simulink library "receiver_sender"  (R2021a)
settings: Solver=ode45  StartTime=0.0  StopTime=10.0  RelTol=1e-3  EnableMultiTasking=on
libraries: dspnetwork x4, etargetslib x4
settings Model: Creator=Adriano  LastModifiedBy=hgu8
settings SolverCC: AlgebraicLoopSolver=TrustRegion
settings DataIOCC: LimitDataPoints=on  SaveFormat=Array  ReturnWorkspaceOutputs=off
settings OptimizationCC: LifeSpan=inf
settings DebuggingCC: UnderspecifiedInitializationDetection=Classic  MergeDetectMultiDrivingBlocksExec=none  SolverPrmCheckMsg=warning  StateNameClashWarn=warning  SFUnexpectedBacktrackingDiag=warning  SFNoUnconditionalDefaultTransitionDiag=warning  SFExecutionAtInitializationDiag=none  SFMachineParentedDataDiag=warning  ArithmeticOperatorsInVariantConditions=warning
settings HardwareCC: ProdBitPerPointer=32  ProdBitPerSizeT=32  ProdBitPerPtrDiffT=32  ProdLargestAtomicFloat=None  ProdIntDivRoundTo=Undefined  ProdEndianess=Unspecified  ProdWordSize=32  ProdHWDeviceType=32-bit Generic
settings ModelReferenceCC: PropagateSignalLabelsOutOfModel=off
settings SFSimCC: SimUseLocalCustomCode=off  CustomCodeUndefinedFunction=UseInterfaceOnly
settings RTWCC: RTWUseLocalCustomCode=off
settings CodeAppCC: StateflowObjectComments=on
settings GRTTargetCC: TargetLangStandard=C89/C90 (ANSI)
settings ConfigComp: CovMetricSettings=dw  CovSaveCumulativeToWorkspaceVar=on  CovSaveSingleToWorkspaceVar=on  CovExternalEMLEnable=off

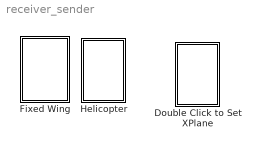
== system receiver_sender ==
  Double Click to Set XPlane : Subsystem
      settings: OpenFcn=selecting_parameters()
  Fixed Wing : Subsystem
  Helicopter : Subsystem

== system receiver_sender/Double Click to Set XPlane ==

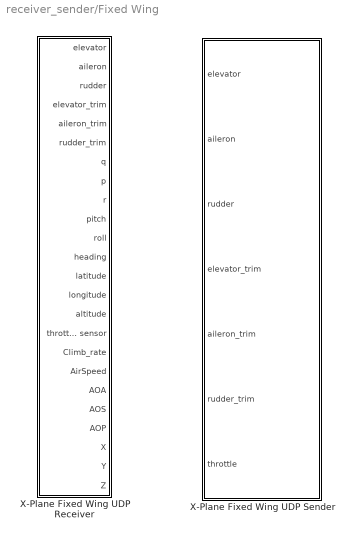
== system receiver_sender/Fixed Wing ==
  X-Plane Fixed Wing UDP Receiver : Subsystem  mask{ip_adress='127.0.0.1', port_number=49004}
      mask prompts: ip_adress "Local IP Adress (default: '127.0.0.1' )"; port_number "Output Port Number (defaut: '49004')"
      mask help: This block is configured to receiver data from a fixed wing aircraft on X-Plane Flight Simulator.
      mask Help: Contact adrianobittar@gmail.com
  X-Plane Fixed Wing UDP Sender : Subsystem  mask{ip_adress='127.0.0.1', port_number=49000}
      mask prompts: ip_adress "Local IP Adress (default: '127.0.0.1' )"; port_number "Output Port Number (defaut: '49000')"
      mask help: This block is configured to send data to a fixed wing aircraft on X-Plane Flight Simulator.
      mask Help: Contact adrianobittar@gmail.com

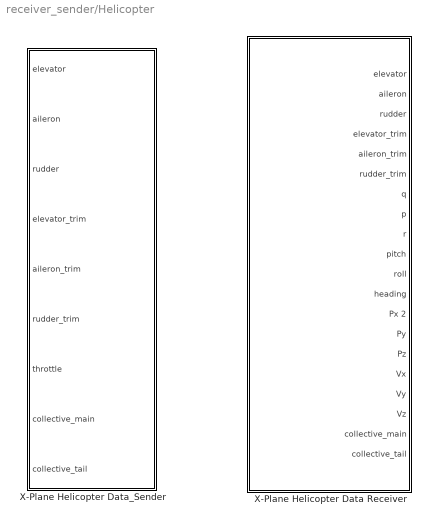
== system receiver_sender/Helicopter ==
  X-Plane Helicopter Data Receiver : Subsystem  AncestorBlock=DU2SRI_Heli_Sim/X-Plane Communication Blockset /X-Plane Data Receiver  mask{ip_adress='127.0.0.1', port_number=49004}
      mask prompts: ip_adress "Local IP Adress (default: '127.0.0.1')"; port_number "Input Port Number (default: '49004')"
      mask help: This block is configured to receive data to an helicopter aircraft on X-Plane Flight Simulator.
      mask Help: Contact adrianobittar@gmail.com
  X-Plane Helicopter Data_Sender : Subsystem  AncestorBlock=DU2SRI_Heli_Sim/X-Plane Communication Blockset /X-Plane Data_Sender  mask{ip_address='127.0.0.1', port_number=49000, max_col_main=12, min_col_main=0, max_col_tail=5, min_col_tail=-5}
      mask prompts: ip_address "Local IP Address (default: '127.0.0.1' )"; port_number "Output Port Number (defaut: '49000')"; max_col_main "Max Angle For Collective Main"; min_col_main "Min Angle For Collective Main"; max_col_tail "Max Angle For Collective Tail"; min_col_tail "Min Angle For Collective Tail"
      mask help: This block is configured to send data to an helicopter aircraft on X-Plane Flight Simulator.
      mask Help: contact adrianobittar@gmail.com

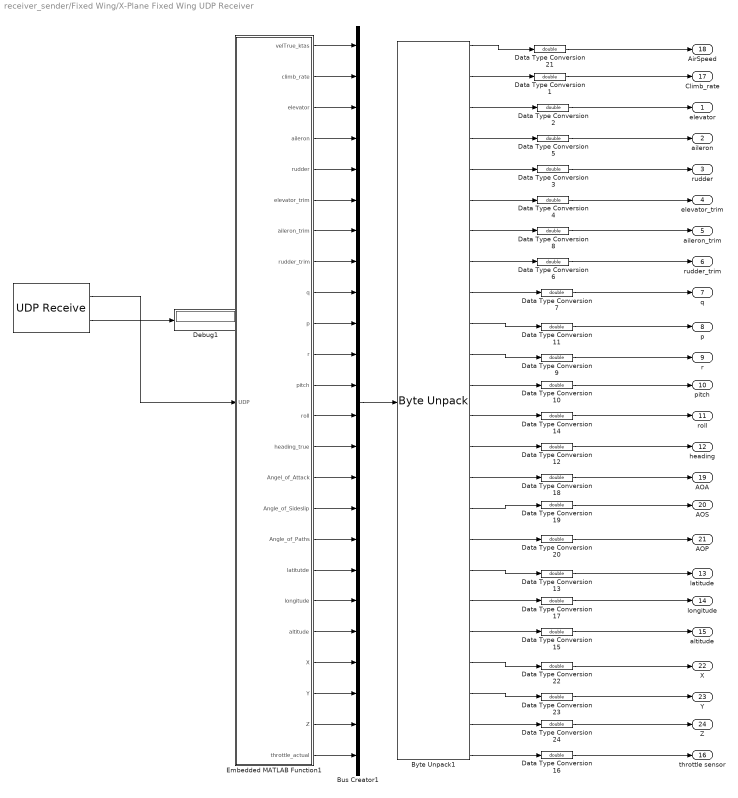
== system receiver_sender/Fixed Wing/X-Plane Fixed Wing UDP Receiver ==
  "    " : dspnetwork/UDP Receive  localURL='0.0.0.0'  localPort=port_number  remoteURL=ip_adress  remotePort=-1  recvBufferSize=8192  dims=500  signalDatatype=uint8  isComplex=off  isVarSize=off  showBlockingTime=on  blockingTime=20  sampletime=0.01  blockPlatform=WINDOWS
  Bus Creator1 : BusCreator  Inputs=24
  Byte Unpack1 : etargetslib/Byte Unpack  dimensions={1,1,1,1,1,1,1,1,1,1,1,1,1,1,1,1,1,1,1,1,1,1,1,1}  datatypes={'single','single','single','single','single','single','single','single','single','single','single','single','single','single','single','single','single','single','single','single','single','single','single','single'}  byteAlign=1
  Data Type Conversion{1..24} (24 alike) : DataTypeConversion  OutDataTypeStr=double  SaturateOnIntegerOverflow=on
  "Debug1 " : Display
  Embedded MATLAB Function1 : MATLAB Function  TreatAsAtomicUnit=on
  "elevator " : Outport
  aileron : Outport  Port=2
  rudder : Outport  Port=3
  elevator_trim : Outport  Port=4
  aileron_trim : Outport  Port=5
  rudder_trim : Outport  Port=6
  q : Outport  Port=7
  p : Outport  Port=8
  r : Outport  Port=9
  pitch : Outport  Port=10
  roll : Outport  Port=11
  heading : Outport  Port=12
  latitude : Outport  Port=13
  longitude : Outport  Port=14
  altitude : Outport  Port=15
  throttle sensor : Outport  Port=16
  Climb_rate : Outport  Port=17
  AirSpeed : Outport  Port=18
  AOA : Outport  Port=19
  AOS : Outport  Port=20
  AOP : Outport  Port=21
  X : Outport  Port=22
  Y : Outport  Port=23
  Z : Outport  Port=24
  wires:
  Data Type Conversion9/1 -> r/1
  Data Type Conversion10/1 -> pitch/1
  "    "/2 -> "Debug1 "/1
  Data Type Conversion21/1 -> AirSpeed/1
  Data Type Conversion1/1 -> Climb_rate/1
  Data Type Conversion2/1 -> "elevator "/1
  Data Type Conversion5/1 -> aileron/1
  Data Type Conversion8/1 -> aileron_trim/1
  Data Type Conversion3/1 -> rudder/1
  Data Type Conversion4/1 -> elevator_trim/1
  Data Type Conversion6/1 -> rudder_trim/1
  Data Type Conversion7/1 -> q/1
  Data Type Conversion12/1 -> heading/1
  Data Type Conversion13/1 -> latitude/1
  Data Type Conversion14/1 -> roll/1
  Data Type Conversion17/1 -> longitude/1
  Data Type Conversion15/1 -> altitude/1
  Data Type Conversion16/1 -> throttle sensor/1
  Data Type Conversion11/1 -> p/1
  Data Type Conversion18/1 -> AOA/1
  Data Type Conversion19/1 -> AOS/1
  Data Type Conversion20/1 -> AOP/1
  Data Type Conversion22/1 -> X/1
  Data Type Conversion23/1 -> Y/1
  Data Type Conversion24/1 -> Z/1
  "    "/1 -> Embedded MATLAB Function1/1(UDP)
  Embedded MATLAB Function1/1(velTrue_ktas) -> Bus Creator1/1
  Embedded MATLAB Function1/2(climb_rate) -> Bus Creator1/2
  Embedded MATLAB Function1/3(elevator) -> Bus Creator1/3
  Embedded MATLAB Function1/4(aileron) -> Bus Creator1/4
  Embedded MATLAB Function1/5(rudder) -> Bus Creator1/5
  Embedded MATLAB Function1/6(elevator_trim) -> Bus Creator1/6
  Embedded MATLAB Function1/7(aileron_trim) -> Bus Creator1/7
  Embedded MATLAB Function1/8(rudder_trim) -> Bus Creator1/8
  Embedded MATLAB Function1/9(q) -> Bus Creator1/9
  Embedded MATLAB Function1/10(p) -> Bus Creator1/10
  Embedded MATLAB Function1/11(r) -> Bus Creator1/11
  Embedded MATLAB Function1/12(pitch) -> Bus Creator1/12
  Embedded MATLAB Function1/13(roll) -> Bus Creator1/13
  Embedded MATLAB Function1/14(heading_true) -> Bus Creator1/14
  Embedded MATLAB Function1/15(Angel_of_Attack) -> Bus Creator1/15
  Embedded MATLAB Function1/16(Angle_of_Sideslip) -> Bus Creator1/16
  Embedded MATLAB Function1/17(Angle_of_Paths) -> Bus Creator1/17
  Embedded MATLAB Function1/18(latitutde) -> Bus Creator1/18
  Embedded MATLAB Function1/19(longitude) -> Bus Creator1/19
  Embedded MATLAB Function1/20(altitude) -> Bus Creator1/20
  Embedded MATLAB Function1/21(X) -> Bus Creator1/21
  Embedded MATLAB Function1/22(Y) -> Bus Creator1/22
  Embedded MATLAB Function1/23(Z) -> Bus Creator1/23
  Embedded MATLAB Function1/24(throttle_actual) -> Bus Creator1/24
  Bus Creator1/1 -> Byte Unpack1/1
  Byte Unpack1/1 -> Data Type Conversion21/1
  Byte Unpack1/2 -> Data Type Conversion1/1
  Byte Unpack1/3 -> Data Type Conversion2/1
  Byte Unpack1/4 -> Data Type Conversion5/1
  Byte Unpack1/5 -> Data Type Conversion3/1
  Byte Unpack1/6 -> Data Type Conversion4/1
  Byte Unpack1/7 -> Data Type Conversion8/1
  Byte Unpack1/8 -> Data Type Conversion6/1
  Byte Unpack1/9 -> Data Type Conversion7/1
  Byte Unpack1/10 -> Data Type Conversion11/1
  Byte Unpack1/11 -> Data Type Conversion9/1
  Byte Unpack1/12 -> Data Type Conversion10/1
  Byte Unpack1/13 -> Data Type Conversion14/1
  Byte Unpack1/14 -> Data Type Conversion12/1
  Byte Unpack1/15 -> Data Type Conversion18/1
  Byte Unpack1/16 -> Data Type Conversion19/1
  Byte Unpack1/17 -> Data Type Conversion20/1
  Byte Unpack1/18 -> Data Type Conversion13/1
  Byte Unpack1/19 -> Data Type Conversion17/1
  Byte Unpack1/20 -> Data Type Conversion15/1
  Byte Unpack1/21 -> Data Type Conversion22/1
  Byte Unpack1/22 -> Data Type Conversion23/1
  Byte Unpack1/23 -> Data Type Conversion24/1
  Byte Unpack1/24 -> Data Type Conversion16/1

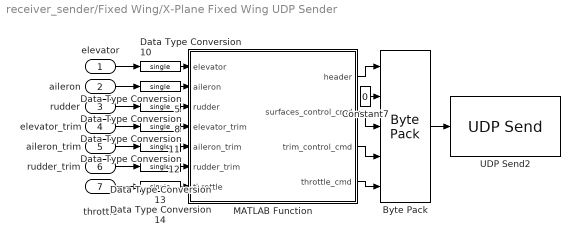
== system receiver_sender/Fixed Wing/X-Plane Fixed Wing UDP Sender ==
  elevator : Inport
  aileron : Inport  Port=2
  rudder : Inport  Port=3
  elevator_trim : Inport  Port=4
  aileron_trim : Inport  Port=5
  rudder_trim : Inport  Port=6
  throttle : Inport  Port=7
  Byte Pack : etargetslib/Byte Pack  datatypes={'single','uint8','single','single','single'}  byteAlign=1
  Constant7 : Constant  Value=0  OutDataTypeStr=uint8
  Data Type Conversion{5,8,10..14} (7 alike) : DataTypeConversion  OutDataTypeStr=single  SaturateOnIntegerOverflow=on
  MATLAB Function : MATLAB Function  TreatAsAtomicUnit=on
  UDP Send2 : dspnetwork/UDP Send  remoteURL=ip_adress  remotePort=port_number  localURL='255.255.255.255'  localPortSource=Automatically determine  localPort=-1  sendBufferSize=8192  sampletime=-1  blockPlatform=HOST  separateLengthPort=0
  wires:
  rudder/1 -> Data Type Conversion8/1
  Constant7/1 -> Byte Pack/2
  Data Type Conversion8/1 -> MATLAB Function/3(rudder)
  throttle/1 -> Data Type Conversion14/1
  Data Type Conversion10/1 -> MATLAB Function/1(elevator)
  Data Type Conversion11/1 -> MATLAB Function/4(elevator_trim)
  aileron/1 -> Data Type Conversion5/1
  elevator/1 -> Data Type Conversion10/1
  MATLAB Function/4(throttle_cmd) -> Byte Pack/5
  Data Type Conversion5/1 -> MATLAB Function/2(aileron)
  Data Type Conversion14/1 -> MATLAB Function/7(throttle)
  MATLAB Function/3(trim_control_cmd) -> Byte Pack/4
  aileron_trim/1 -> Data Type Conversion12/1
  Data Type Conversion13/1 -> MATLAB Function/6(rudder_trim)
  Data Type Conversion12/1 -> MATLAB Function/5(aileron_trim)
  MATLAB Function/1(header) -> Byte Pack/1
  elevator_trim/1 -> Data Type Conversion11/1
  Byte Pack/1 -> UDP Send2/1
  MATLAB Function/2(surfaces_control_cmd) -> Byte Pack/3
  rudder_trim/1 -> Data Type Conversion13/1

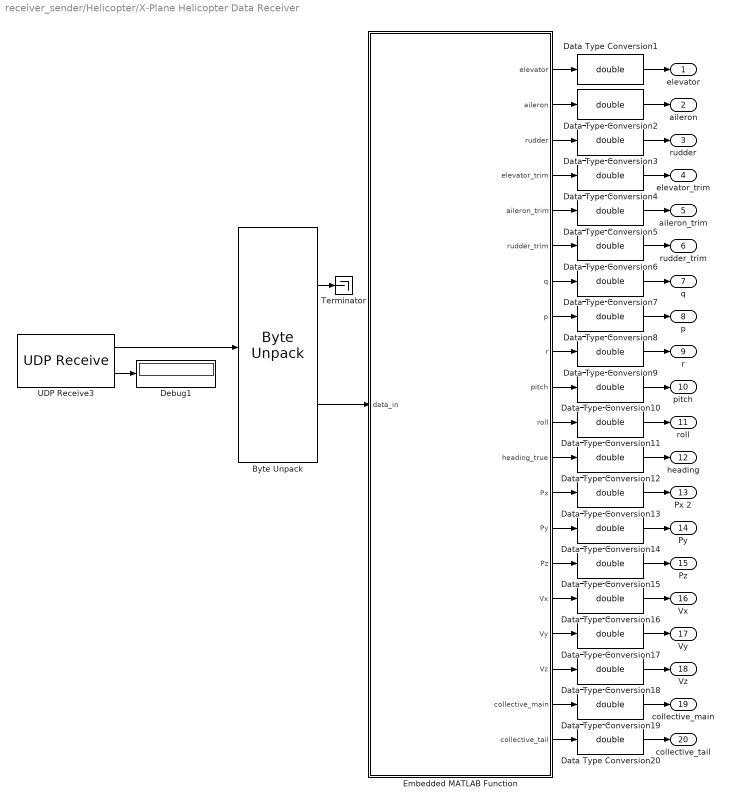
== system receiver_sender/Helicopter/X-Plane Helicopter Data Receiver ==
  Byte Unpack : etargetslib/Byte Unpack  dimensions={5,[9,6]}  datatypes={'uint8','single'}  byteAlign=1
  Data Type Conversion{1..20} (20 alike) : DataTypeConversion  OutDataTypeStr=double  SaturateOnIntegerOverflow=on
  "Debug1 " : Display
  Embedded MATLAB Function : MATLAB Function  TreatAsAtomicUnit=on
  Terminator : Terminator
  UDP Receive3 : dspnetwork/UDP Receive  localURL='0.0.0.0'  localPort=port_number  remoteURL=ip_adress  remotePort=-1  recvBufferSize=8192  dims=221  signalDatatype=uint8  isComplex=off  isVarSize=off  showBlockingTime=on  blockingTime=20  sampletime=0  blockPlatform=WINDOWS
  "elevator " : Outport
  aileron : Outport  Port=2
  rudder : Outport  Port=3
  elevator_trim : Outport  Port=4
  aileron_trim : Outport  Port=5
  rudder_trim : Outport  Port=6
  q : Outport  Port=7
  p : Outport  Port=8
  r : Outport  Port=9
  pitch : Outport  Port=10
  roll : Outport  Port=11
  heading : Outport  Port=12
  Px 2 : Outport  Port=13
  Py : Outport  Port=14
  Pz : Outport  Port=15
  Vx : Outport  Port=16
  Vy : Outport  Port=17
  Vz : Outport  Port=18
  collective_main : Outport  Port=19
  collective_tail : Outport  Port=20
  wires:
  Embedded MATLAB Function/10(pitch) -> Data Type Conversion10/1
  Data Type Conversion8/1 -> p/1
  Data Type Conversion13/1 -> Px 2/1
  Data Type Conversion1/1 -> "elevator "/1
  Byte Unpack/1 -> Terminator/1
  UDP Receive3/2 -> "Debug1 "/1
  Data Type Conversion4/1 -> elevator_trim/1
  Embedded MATLAB Function/8(p) -> Data Type Conversion8/1
  Data Type Conversion12/1 -> heading/1
  Embedded MATLAB Function/11(roll) -> Data Type Conversion11/1
  Embedded MATLAB Function/1(elevator) -> Data Type Conversion1/1
  Data Type Conversion10/1 -> pitch/1
  Embedded MATLAB Function/3(rudder) -> Data Type Conversion3/1
  Data Type Conversion2/1 -> aileron/1
  Data Type Conversion6/1 -> rudder_trim/1
  UDP Receive3/1 -> Byte Unpack/1
  Data Type Conversion9/1 -> r/1
  Data Type Conversion11/1 -> roll/1
  Embedded MATLAB Function/7(q) -> Data Type Conversion7/1
  Embedded MATLAB Function/18(Vz) -> Data Type Conversion18/1
  Data Type Conversion18/1 -> Vz/1
  Data Type Conversion5/1 -> aileron_trim/1
  Data Type Conversion15/1 -> Pz/1
  Data Type Conversion19/1 -> collective_main/1
  Embedded MATLAB Function/14(Py) -> Data Type Conversion14/1
  Embedded MATLAB Function/5(aileron_trim) -> Data Type Conversion5/1
  Embedded MATLAB Function/19(collective_main) -> Data Type Conversion19/1
  Embedded MATLAB Function/6(rudder_trim) -> Data Type Conversion6/1
  Embedded MATLAB Function/20(collective_tail) -> Data Type Conversion20/1
  Data Type Conversion16/1 -> Vx/1
  Embedded MATLAB Function/12(heading_true) -> Data Type Conversion12/1
  Embedded MATLAB Function/13(Px) -> Data Type Conversion13/1
  Data Type Conversion17/1 -> Vy/1
  Embedded MATLAB Function/4(elevator_trim) -> Data Type Conversion4/1
  Data Type Conversion14/1 -> Py/1
  Embedded MATLAB Function/17(Vy) -> Data Type Conversion17/1
  Embedded MATLAB Function/2(aileron) -> Data Type Conversion2/1
  Embedded MATLAB Function/16(Vx) -> Data Type Conversion16/1
  Data Type Conversion3/1 -> rudder/1
  Embedded MATLAB Function/15(Pz) -> Data Type Conversion15/1
  Embedded MATLAB Function/9(r) -> Data Type Conversion9/1
  Data Type Conversion7/1 -> q/1
  Data Type Conversion20/1 -> collective_tail/1
  Byte Unpack/2 -> Embedded MATLAB Function/1(data_in)

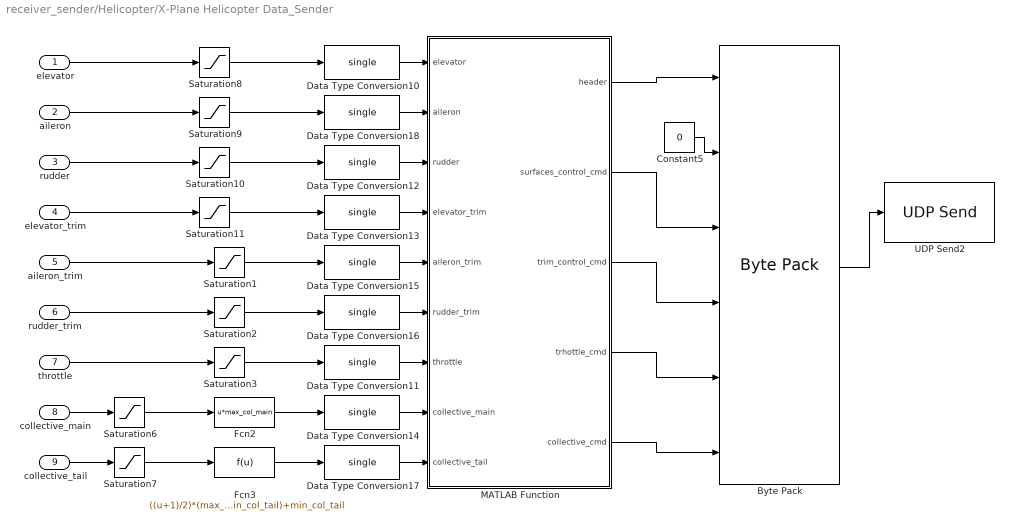
== system receiver_sender/Helicopter/X-Plane Helicopter Data_Sender ==
  elevator : Inport
  aileron : Inport  Port=2
  rudder : Inport  Port=3
  elevator_trim : Inport  Port=4
  aileron_trim : Inport  Port=5
  rudder_trim : Inport  Port=6
  throttle : Inport  Port=7
  collective_main : Inport  Port=8
  collective_tail : Inport  Port=9
  Byte Pack : etargetslib/Byte Pack  datatypes={'single','uint8','single','single','single','single'}  byteAlign=1
  Constant5 : Constant  Value=0  OutDataTypeStr=uint8
  Data Type Conversion{10..18} (9 alike) : DataTypeConversion  OutDataTypeStr=single  SaturateOnIntegerOverflow=on
  Fcn2 : Fcn  Expr=u*max_col_main
  Fcn3 : Fcn  Expr=((u+1)/2)*(max_col_tail-min_col_tail)+min_col_tail
  MATLAB Function : MATLAB Function  TreatAsAtomicUnit=on
  Saturation{1..3,6..11} (9 alike) : Saturate  UpperLimit=+1  LowerLimit=-1
  UDP Send2 : dspnetwork/UDP Send  remoteURL=ip_address  remotePort=port_number  localURL='255.255.255.255'  localPortSource=Automatically determine  localPort=-1  sendBufferSize=8192  sampletime=-1  blockPlatform=HOST  separateLengthPort=0
  wires:
  Saturation8/1 -> Data Type Conversion10/1
  Data Type Conversion18/1 -> MATLAB Function/2(aileron)
  Constant5/1 -> Byte Pack/2
  MATLAB Function/5(collective_cmd) -> Byte Pack/6
  MATLAB Function/4(trhottle_cmd) -> Byte Pack/5
  MATLAB Function/3(trim_control_cmd) -> Byte Pack/4
  MATLAB Function/2(surfaces_control_cmd) -> Byte Pack/3
  MATLAB Function/1(header) -> Byte Pack/1
  Byte Pack/1 -> UDP Send2/1
  Data Type Conversion17/1 -> MATLAB Function/9(collective_tail)
  Data Type Conversion14/1 -> MATLAB Function/8(collective_main)
  Data Type Conversion11/1 -> MATLAB Function/7(throttle)
  Data Type Conversion16/1 -> MATLAB Function/6(rudder_trim)
  Data Type Conversion15/1 -> MATLAB Function/5(aileron_trim)
  Data Type Conversion13/1 -> MATLAB Function/4(elevator_trim)
  Data Type Conversion12/1 -> MATLAB Function/3(rudder)
  Data Type Conversion10/1 -> MATLAB Function/1(elevator)
  Saturation10/1 -> Data Type Conversion12/1
  Saturation11/1 -> Data Type Conversion13/1
  Saturation9/1 -> Data Type Conversion18/1
  Saturation7/1 -> Fcn3/1
  Saturation6/1 -> Fcn2/1
  collective_main/1 -> Saturation6/1
  collective_tail/1 -> Saturation7/1
  Saturation3/1 -> Data Type Conversion11/1
  elevator_trim/1 -> Saturation11/1
  Saturation1/1 -> Data Type Conversion15/1
  aileron/1 -> Saturation9/1
  Saturation2/1 -> Data Type Conversion16/1
  elevator/1 -> Saturation8/1
  Fcn2/1 -> Data Type Conversion14/1
  rudder/1 -> Saturation10/1
  aileron_trim/1 -> Saturation1/1
  rudder_trim/1 -> Saturation2/1
  throttle/1 -> Saturation3/1
  Fcn3/1 -> Data Type Conversion17/1

== matlab function receiver_sender/Helicopter/X-Plane Helicopter Data Receiver/Embedded MATLAB Function ==
  data: data_in input; elevator output; aileron output; rudder output; elevator_trim output; aileron_trim output; rudder_trim output; q output; p output; r output; pitch output; roll output; heading_true output; Px output; Py output; Pz output; Vx output; Vy output; Vz output; collective_main output; collective_tail output
function [elevator, aileron, rudder, elevator_trim, aileron_trim, rudder_trim, q,p,r, pitch, roll, heading_true, Px, Py, Pz, Vx, Vy, Vz, collective_main, collective_tail]   = fcn(data_in)
% This block supports the Embedded MATLAB subset.
% See the help menu for details. 

elevator = data_in(2,1);
aileron = data_in(3,1);
rudder= data_in(4,1);


elevator_trim= data_in(2,2);
aileron_trim= data_in(3,2);
rudder_trim= data_in(4,2);

q= data_in(2,3);
p= data_in(3,3);
r= data_in(4,3);

pitch= data_in(2,4);
roll= data_in(3,4);
heading_true= data_in(4,4);

Px= data_in(2,5);
Py= data_in(3,5);
Pz= data_in(4,5);
Vx= data_in(5,5);
Vy= data_in(6,5);
Vz= data_in(7,5);

collective_main= data_in(2,6);
collective_tail= data_in(3,6);

== matlab function receiver_sender/Fixed Wing/X-Plane Fixed Wing UDP Receiver/Embedded MATLAB Function1 ==
  data: velTrue_ktas output; climb_rate output; UDP input; elevator output; aileron output; rudder output; elevator_trim output; aileron_trim output; rudder_trim output; q output; p output; r output; pitch output; roll output; heading_true output; Angel_of_Attack output; Angle_of_Sideslip output; Angle_of_Paths output; latitutde output; longitude output; altitude output; X output; Y output; Z output; throttle_actual output
% X-PLANE: Channels 3,4,8,13,16,17,18,20,21,26
%---------------------------------------------------------------------------------------------------
% flight_con = [elev ailrn ruddr];                         %flight controls
% attitude = [pitch roll hding_true hding_mag];            %pitch,roll,yaw
% location = [lat lon alt_msl alt_agl];                    &x,y,z
% %latitude,longitude,altitude[deg],[ftmsl],[ftagl](mean sea level,actual ground level)
% control algorithm needs x-y-z axis position,forward speed,FLIGHT path
% angle, Yaw angle, Angle of sideslipe
% Angel of attack,sideslip,&paths                          %
%---------------------------------------------------------------------------------------------------
function [velTrue_ktas, climb_rate,elevator, aileron, rudder, elevator_trim, aileron_trim, rudder_trim, q,p,r, pitch, roll, heading_true, Angel_of_Attack, Angle_of_Sideslip ,Angle_of_Paths ,latitutde, longitude, altitude, X, Y, Z, throttle_actual] = fcn(UDP)

%we do not need the DATA header, which are the first 5 bytes
UDP = UDP(6:end);

%we cut the datagram in channels, each containing 36 bytes, 4 for the
%channel number, and 4 for each of the 8 entries.
CH3 = UDP(1:36);
CH4 = UDP(37:72);
CH8 = UDP(73:108);
CH13 = UDP(109:144);
CH16 = UDP(145:180);
CH17 = UDP(181:216);
CH18 = UDP(217:252);
CH20 = UDP(253:288);
CH21 = UDP(289:324);
CH26 = UDP(325:360);

%-------------
% At last we extract each entry from their channel and output them.
%elev = Channel_to_single(CH11,1);
%ailrn = Channel_to_single(CH11,2);
%ruddr = Channel_to_single(CH11,3);

velTrue_ktas = Channel_to_single(CH3,6);

climb_rate = Channel_to_single(CH4,1);
%VVI, fpm The aircraft’s current vertical velocity, 
%in feet per minute. If everything is working as it should, 
%this is normal to the local horizon under the aircraft.

elevator = Channel_to_single(CH8,1);
aileron = Channel_to_single(CH8,2);
rudder= Channel_to_single(CH8,3);

elevator_trim= Channel_to_single(CH13,1);
aileron_trim= Channel_to_single(CH13,2);
rudder_trim= Channel_to_single(CH13,3);

q= Channel_to_single(CH16,1);
p= Channel_to_single(CH16,2);
r= Channel_to_single(CH16,3);

pitch= Channel_to_single(CH17,1);
roll= Channel_to_single(CH17,2);
heading_true= Channel_to_single(CH17,3);

%Angle_of_Attack is heading angle which is from hpath channel 3
Angel_of_Attack = Channel_to_single(CH18,3);
Angle_of_Sideslip = Channel_to_single(CH18,2);
Angle_of_Paths = Channel_to_single(CH18,4);
%Angle_of_Paths is FlightPathAngle which is from hpath channel 4

latitutde= Channel_to_single(CH20,1);
longitude= Channel_to_single(CH20,2);
altitude= Channel_to_single(CH20,3);

X = Channel_to_single(CH21,1);
Y = Channel_to_single(CH21,2);
Z = Channel_to_single(CH21,3);


throttle_actual = Channel_to_single(CH26,1);


%--------------
end

function [single] = Channel_to_single(CH,data_pos)

start_byte = 1+4*data_pos;
stop_byte = start_byte+3;
single = CH(start_byte:stop_byte);

end

== matlab function receiver_sender/Helicopter/X-Plane Helicopter Data_Sender/MATLAB Function ==
  data: elevator input single size=1; aileron input; rudder input; elevator_trim input; aileron_trim input; rudder_trim input; throttle input; collective_main input; collective_tail input; header output single size=1; surfaces_control_cmd output single size=[1 18]; trim_control_cmd output single size=[1 18]; trhottle_cmd output single size=[1 9]; collective_cmd output single size=[1 9]
function [header, surfaces_control_cmd,trim_control_cmd,trhottle_cmd,collective_cmd]  = fcn(elevator, aileron, rudder, elevator_trim, aileron_trim, rudder_trim, throttle, collective_main, collective_tail)
% This block supports the Embedded MATLAB subset.
% See the help menu for details. 

header = typecast(uint8([uint8(68) uint8(65) uint8(84) uint8(65)]), 'single');




No_Comand = single(-999);

Surface_header = typecast(uint8([uint8(8) uint8(0) uint8(0) uint8(0)]), 'single');

surfaces_control_cmd = [Surface_header elevator aileron rudder No_Comand No_Comand No_Comand No_Comand No_Comand Surface_header No_Comand No_Comand No_Comand No_Comand No_Comand No_Comand No_Comand No_Comand];

Trim_header = typecast(uint8([uint8(13) uint8(0) uint8(0) uint8(0)]), 'single');


trim_control_cmd = [ Trim_header elevator_trim aileron_trim rudder_trim No_Comand No_Comand No_Comand No_Comand No_Comand Trim_header No_Comand No_Comand No_Comand No_Comand No_Comand No_Comand No_Comand No_Comand];

Throttle_header = typecast(uint8([uint8(25) uint8(0) uint8(0) uint8(0)]), 'single');
trhottle_cmd = [Throttle_header throttle No_Comand No_Comand No_Comand No_Comand No_Comand No_Comand No_Comand];

Collective_header = typecast(uint8([uint8(39) uint8(0) uint8(0) uint8(0)]), 'single');

collective_cmd = [ Collective_header collective_main collective_tail No_Comand No_Comand No_Comand No_Comand No_Comand No_Comand];
%data_out = [surfaces_control_cmd trim_control_cmd trhottle_cmd collective_cmd];


% Actuadors_Out[0] = 68;
% Actuadors_Out[1] = 65;
% Actuadors_Out[2] = 84;
% Actuadors_Out[3] = 65;
% Actuadors_Out[4] = 48;//26;
% aileron = data_in(3,1);
% rudder= data_in(4,1);
% 
% 
% elevator_trim= data_in(2,2);
% aileron_trim= data_in(3,2);
% rudder_trim= data_in(4,2);
% 
% q= data_in(2,3);
% p= data_in(3,3);
% r= data_in(4,3);
% 
% pitch= data_in(2,4);
% roll= data_in(3,4);
% heading_true= data_in(4,4);
% 
% Px= data_in(2,5);
% Py= data_in(3,5);
% Pz= data_in(4,5);
% Vx= data_in(5,5);
% Vy= data_in(6,5);
% Vz= data_in(7,5);
% 
% collective_main= data_in(2,6);
% collective_tail= data_in(3,6);

== matlab function receiver_sender/Fixed Wing/X-Plane Fixed Wing UDP Sender/MATLAB Function ==
  data: elevator input single size=1; aileron input; rudder input; elevator_trim input; aileron_trim input; rudder_trim input; throttle input; header output single size=1; surfaces_control_cmd output single size=[1 18]; trim_control_cmd output single size=[1 18]; throttle_cmd output size=[1 18]
function [header, surfaces_control_cmd,trim_control_cmd, throttle_cmd]  = fcn(elevator, aileron, rudder, elevator_trim, aileron_trim, rudder_trim, throttle)
% This block supports the Embedded MATLAB subset.
% See the help menu for details. 

header = typecast(uint8([uint8(68) uint8(65) uint8(84) uint8(65)]), 'single');



No_Comand = single(-999);

Surface_header = typecast(uint8([uint8(8) uint8(0) uint8(0) uint8(0)]), 'single');

surfaces_control_cmd = [Surface_header elevator aileron rudder No_Comand No_Comand No_Comand No_Comand No_Comand Surface_header No_Comand No_Comand No_Comand No_Comand No_Comand No_Comand No_Comand No_Comand];

Trim_header = typecast(uint8([uint8(13) uint8(0) uint8(0) uint8(0)]), 'single');


trim_control_cmd = [ Trim_header elevator_trim aileron_trim rudder_trim No_Comand No_Comand No_Comand No_Comand No_Comand Trim_header No_Comand No_Comand No_Comand No_Comand No_Comand No_Comand No_Comand No_Comand];

Throttle_header = typecast(uint8([uint8(25) uint8(0) uint8(0) uint8(0)]), 'single');
throttle_cmd = [Throttle_header throttle No_Comand No_Comand No_Comand No_Comand No_Comand No_Comand No_Comand Throttle_header No_Comand No_Comand No_Comand No_Comand No_Comand No_Comand No_Comand No_Comand];




% Actuadors_Out[0] = 68;
% Actuadors_Out[1] = 65;
% Actuadors_Out[2] = 84;
% Actuadors_Out[3] = 65;
% Actuadors_Out[4] = 48;//26;
% aileron = data_in(3,1);
% rudder= data_in(4,1);
% 
% 
% elevator_trim= data_in(2,2);
% aileron_trim= data_in(3,2);
% rudder_trim= data_in(4,2);
% 
% q= data_in(2,3);
% p= data_in(3,3);
% r= data_in(4,3);
% 
% pitch= data_in(2,4);
% roll= data_in(3,4);
% heading_true= data_in(4,4);
% 
% Px= data_in(2,5);
% Py= data_in(3,5);
% Pz= data_in(4,5);
% Vx= data_in(5,5);
% Vy= data_in(6,5);
% Vz= data_in(7,5);
% 
% collective_main= data_in(2,6);
% collective_tail= data_in(3,6);
